simulink library "gasLibrary"  (R2019a)
settings: Solver=VariableStepAuto  StartTime=0.0  StopTime=10.0  RelTol=1e-3
values from neighbouring files (symbols this model uses):
  loadControlFlag = "on"    [gas_v1.m]
  loadState = "on"    [ColoradoGasModel.m]    (also in compressorTest.m = 'on'; experiment1.m = 'on'; experiment2.m = 'on'; experiment3.m = 'on')
  shutOffDuration = 3600    [ColoradoGasModel.m]
  shutOffPoint = 600    [ColoradoGasModel.m]
undefined symbols (not defined in the file or in its folder): f, powerSetPort, pressureSendPort, tempSendPort
libraries: fl_lib x48, nesl_utility x18, $bdroot x13, instrumentlib x5
settings Model: Creator=dzimm  LastModifiedBy=brandt

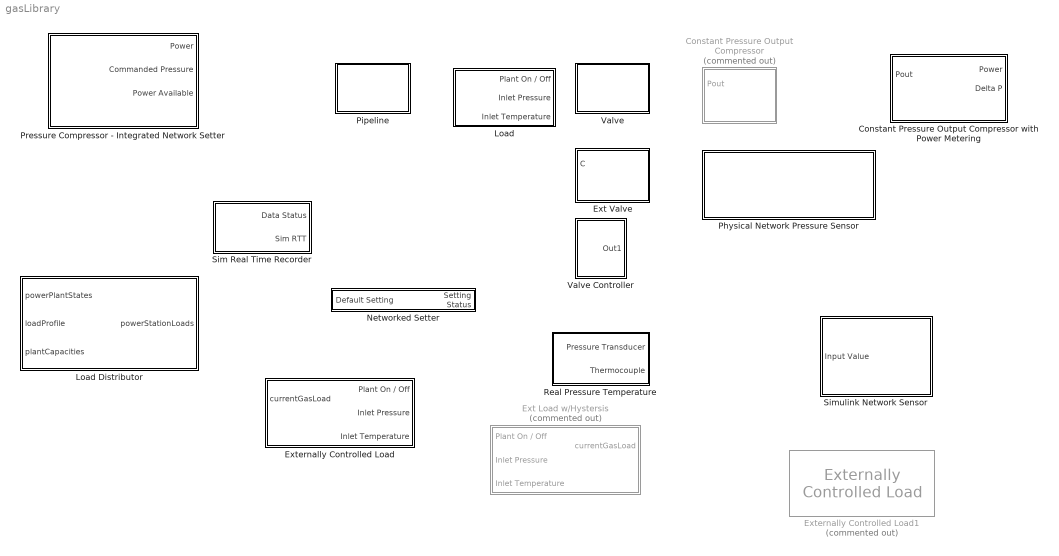
== system gasLibrary ==
  Constant Pressure Output Compressor : Subsystem  Commented=on  mask{xferNum=1, xferDen=[1800 1], delaySeconds=1, efficiency=0.3}
      mask prompts: xferNum "Plant Transfer Function Numerator (vector)"; xferDen "Plant Transfer Function Denominator (vector)"; delaySeconds "Response Delay (s)"; efficiency "Full Efficiency (-)"
  Constant Pressure Output Compressor with Power Metering : Subsystem  AncestorBlock=gasLibrary/Constant Pressure Output Compressor  mask{xferNum=1, xferDen=[1800 1], delaySeconds=1, efficiency=0.3, Numerator=[25]}
      mask prompts: xferNum "Plant Transfer Function Numerator (vector)"; xferDen "Plant Transfer Function Denominator (vector)"; delaySeconds "Response Delay (s)"; efficiency "Full Efficiency (-)"; Numerator "PSI Compression Ratio"
      mask TypeOptions Numerator: Power Transfer Function/Numerator
  Ext Load w/Hystersis : Subsystem  Commented=on  AncestorBlock=gasLibrary/Externally Controlled Load  mask{loadRow=0, loadState=loadState, pressureSendPort=8000, tempSendPort=9000, shutoff_duration=3600, shutoff_point=600}
      mask prompts: loadRow "Load Parameters (table row)"; loadState "Load Simulation Control ('on','off','initial')"; pressureSendPort "Pressure send port:"; tempSendPort "Temperature send port:"; shutoff_duration "Shut Off Duration (Seconds)"; shutoff_point "Shut Off Point (PSI)"
      mask init:
      | if(isempty(loadRow)||isnumeric(loadRow))
      |     loadName="Load";
      |     gasTime=[0 1e6]';
      |     gasLoad=[0 0]';
      |     textColor='red';
      |     pNominal=300;
      |     pCutoff=150;
      | else
      |     loadName=loadRow.Name;
      |     t=loadRow.Time{1};
      |     g=loadRow.Load{1};
      |     pNominal=loadRow.NominalPressure;
      |     pCutoff=loadRow.PressureCutoff;
      |     stopTime=loadRow.Time{1}(length(loadRow.Time{1}));
      |     switch(lower(loadState))
      |         case "on"
      | %             gasTime=t(:);
      | %             gasLoad=g(:);
      |             gasTime=[0 1e6]';
      |             gasLoad=[0 0]';
      |             textColor='green';
      |             loadFlag=[stopTime 1];
      |         case "off"
      |             textColor='red';
      |             gasTime=[0 1e6]';
      |             gasLoad=[0 0]';
      |             loadFlag=[stopTime 2];
      |         case "initial"
      |             textColor='blue';
      |             gasTime=[0 24*3600 1e6 ]';     % ramp gas on over one day
      |             gasLoad=[0 0       5   ]';     % gas ends at initial value
      |             loadFlag=[stopTime 3];
      |         otherwise
      |             fprintf("Cannot initialize\n");
      |             textColor='green';
      |     end
      | end
      mask TypeOptions pressureSendPort: Load Pressure UDP Send/Port
      mask TypeOptions tempSendPort: Load Temperature UDP Send/Port
      mask TypeOptions shutoff_duration: Pressure Shutoff/shutoff_duration
      mask TypeOptions shutoff_point: Pressure Shutoff/shutoff_point
      mask Display:
      | % tMax=max([gasTime(end)]);
      | set_param(gcb,'Name',loadName);
      | % color(textColor);
      | % text(0.1,0.8,sprintf("%s / %2.1f kg/s",loadState,max(gasLoad)))
      | % plot([0.2 0.8],[0.1 0.1]);
      | % plot([0.2 0.2],[0.1 0.6]);
      | % plot(gasTime/tMax*0.6+0.2,gasLoad/max(gasLoad)*0.5+0.1);
  Ext Valve : Subsystem  AncestorBlock=gasLibrary/Valve  mask{valveRow=[], valveState="on"}
      mask prompts: valveRow "Valve Control (table row)"; valveState "Valve Simulation Control ('on' 'off' 'initial')"
      mask init:
      | if(isempty(valveRow)||isnumeric(valveRow))
      |     valveName="Valve";
      |     valveTime=[0 1e6]';
      |     valveSetting=[0 0]';
      |     D=20;           % size of the valve
      |     Dmax=D-1;       % maximum port opening
      |     textColor='red';
      | else
      |     valveName=valveRow.Name;
      |     t=valveRow.Time{1};
      |     g=valveRow.State{1};
      |     D=valveRow.PortDiameter;
      |     Dmax=valveRow.MaxValveDiameter;
      |     switch(lower(valveState))
      |         case "on"
      |             valveTime=t(:);
      |             valveSetting=g(:);
      |             textColor='green';
      |         case "off"
      |             valveTime=[0 1e6]';
      |             valveSetting=[1 1]';
      |             textColor='red';
      |         case "initial"
      |             valveTime=[0 1e6 ]';   % ramp gas on over one day
      |             valveSetting=[g(1)    g(1)]';     % gas ends at initial value
      |             textColor='blue';
      |         otherwise
      |             fprintf("Cannot initialize\n");
      |             textColor='green';
      |     end
      | end
      mask Display:
      | set_param(gcb,'Name',valveName);
      | color(textColor);
      | if(valveState=="off")
      |     vLabel="bypass";
      | else
      |     vLabel="active";
      | end
      | text(0.1,0.8,sprintf("%s (%1d in)",vLabel,D))
      | plot([0.2 0.9],[0.3 0.3]);
      | plot([0.2 0.2],[0.1 0.6]);
      | plot(valveTime/max(valveTime)*0.65+0.2,double(valveSetting)*0.4+0.15);
  Externally Controlled Load : Subsystem  AncestorBlock=gasLibrary/Externally Controlled Load  mask{loadRow=0, loadState=loadState, pressureSendPort=8007, tempSendPort=8008, shutoff_duration=shutOffDuration, shutoff_point=shutOffPoint}
      mask prompts: loadRow "Load Parameters (table row)"; loadState "Load Simulation Control ('on','off','initial')"; pressureSendPort "Pressure send port:"; tempSendPort "Temperature send port:"; shutoff_duration "Shut Off Duration (Seconds)"; shutoff_point "Shut Off Point (PSI)"
      mask init: same as gasLibrary/Ext Load w/Hystersis
      mask TypeOptions pressureSendPort: Load Pressure UDP Send/Port
      mask TypeOptions tempSendPort: Load Temperature UDP Send/Port
      mask TypeOptions shutoff_duration: Pressure Shutoff/shutoff_duration
      mask TypeOptions shutoff_point: Pressure Shutoff/shutoff_point
      mask Display:
      | % tMax=max([gasTime(end)]);
      | set_param(gcb,'Name',loadName);
      | % color(textColor);
      | % text(0.1,0.8,sprintf("%s / %2.1f kg/s",loadState,max(gasLoad)))
      | % plot([0.2 0.8],[0.1 0.1]);
      | % plot([0.2 0.2],[0.1 0.6]);
      | % plot(gasTime/tMax*0.6+0.2,gasLoad/max(gasLoad)*0.5+0.1);
  Externally Controlled Load1 : $bdroot/Externally Controlled Load  Commented=on  loadRow=0  loadState=loadState  pressureSendPort=8007  tempSendPort=8008  shutoff_duration=shutoff_duration  shutoff_point=shutoff_point
  Load : Subsystem  mask{loadRow=0, loadState=loadControlFlag}
      mask prompts: loadRow "Load Parameters (table row)"; loadState "Load Simulation Control ('on','off','initial')"
      mask init:
      | if(isempty(loadRow)||isnumeric(loadRow))
      |     loadName="Load";
      |     gasTime=[0 1e6]';
      |     gasLoad=[0 0]';
      |     textColor='red';
      |     pNominal=300;
      |     pCutoff=150;
      | else
      |     loadName=loadRow.Name;
      |     t=loadRow.Time{1};
      |     g=loadRow.Load{1};
      |     pNominal=loadRow.NominalPressure;
      |     pCutoff=loadRow.PressureCutoff;
      |     switch(lower(loadState))
      |         case "on"
      |             gasTime=t(:);
      |             gasLoad=g(:);
      |             textColor='green';
      |         case "off"
      |             gasTime=[0 1e6]';
      |             gasLoad=[0 0]';
      |             textColor='red';
      |         case "initial"
      |             gasTime=[0 24*3600 1e6 ]';   % ramp gas on over one day
      |             gasLoad=[0 g(1)    g(1)]';     % gas ends at initial value
      |             textColor='blue';
      |         otherwise
      |             fprintf("Cannot initialize\n");
      |             textColor='green';
      |     end
      | end
      mask Display:
      | tMax=max([gasTime(end)]);
      | set_param(gcb,'Name',loadName);
      | color(textColor);
      | text(0.1,0.8,sprintf("%s / %2.1f kg/s",loadState,max(gasLoad)))
      | plot([0.2 0.8],[0.1 0.1]);
      | plot([0.2 0.2],[0.1 0.6]);
      | plot(gasTime/tMax*0.6+0.2,gasLoad/max(gasLoad)*0.5+0.1);
  Load Distributor : MATLAB Function  TreatAsAtomicUnit=on
  Networked Setter : Subsystem  mask{LocalPort=9090}
      mask prompts: LocalPort "Local port:"
      mask TypeOptions LocalPort: UDP Receive/LocalPort
  "Physical Network Pressure Sensor " : Subsystem
  Pipeline : Subsystem  mask{pipeRow=[]}
      mask prompts: pipeRow "Pipeilne Configuration (table row)"
      mask init:
      | if(isempty(pipeRow))
      |     pipeName="Pipeline";
      |     D=24;
      |     L=50;
      |     Pstart=300;
      | else
      |     pipeName=pipeRow.Name;
      |     D=pipeRow.DiameterInch;
      |     L=pipeRow.LengthMiles;
      |     Pstart=pipeRow.StartPressurePSI;
      | end
      mask Display:
      | fprintf('%1d"\n%1d miles\n%1d psi',D,L,Pstart)
      | set_param(gcb,'Name',pipeName)
  Pressure Compressor - Integrated Network Setter : Subsystem  AncestorBlock=gasLibrary/Constant Pressure Output Compressor  mask{xferNum=1, xferDen=[1800 1], delaySeconds=1, efficiency=0.3, pOutDefault=800, setterPort=9090, powerSetPort=powerSetPort, pressurePort=pressureSendPort, tempPort=tempSendPort}
      mask prompts: xferNum "Plant Transfer Function Numerator (vector)"; xferDen "Plant Transfer Function Denominator (vector)"; delaySeconds "Response Delay (s)"; efficiency "Full Efficiency (-)"; pOutDefault "Nominal Pressure:"; setterPort "Pressure setter port:"; powerSetPort "Power setter port:"; pressurePort "Pressure Port:"; tempPort "Temperature Port:"
      mask TypeOptions pOutDefault: Default POut/Value
      mask TypeOptions setterPort: Networked Setter/LocalPort
      mask TypeOptions powerSetPort: Max Power Setter/LocalPort
      mask TypeOptions pressurePort: Compressor Pressure UDP Send/Port
      mask TypeOptions tempPort: Compressor Temp UDP Send/Port
  Real Pressure Temperature : Subsystem  AncestorBlock=gasLibrary/Physical to Real Pressure Temperature
  Sim Real Time Recorder : Subsystem  mask{sendPort=6068, recPort=6065}
      mask prompts: sendPort "Send Port:"; recPort "Receive port:"
      mask TypeOptions sendPort: UDP Send/Port
      mask TypeOptions recPort: UDP Receive/LocalPort
  Simulink Network Sensor : Subsystem  mask{Port=7070}
      mask prompts: Port "Remote Port:"
      mask TypeOptions Port: UDP Send/Port
  Valve : Subsystem  mask{valveRow=[], valveState="on"}
      mask prompts: valveRow "Valve Control (table row)"; valveState "Valve Simulation Control ('on' 'off' 'initial')"
      mask init: same as gasLibrary/Ext Valve
      mask Display:
      | set_param(gcb,'Name',valveName);
      | color(textColor);
      | if(valveState=="off")
      |     vLabel="bypass";
      | else
      |     vLabel="active";
      | end
      | text(0.1,0.8,sprintf("%s (%1d in)",vLabel,D))
      | plot([0.2 0.9],[0.3 0.3]);
      | plot([0.2 0.2],[0.1 0.6]);
      | plot(valveTime/max(valveTime)*0.65+0.2,double(valveSetting)*0.4+0.15);
  Valve Controller : Subsystem

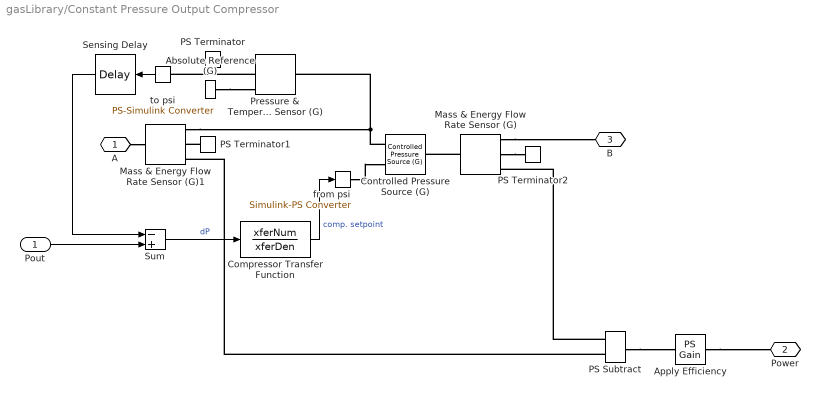
== system gasLibrary/Constant Pressure Output Compressor ==
  Pout : Inport
  Absolute Reference (G) : fl_lib/Gas/Elements/Absolute Reference (G)
      settings: SourceProductName=Simscape  SourceProductBaseCode=SS
  Apply Efficiency : fl_lib/Physical Signals/Functions/PS Gain  gain=1/efficiency
  Compressor Transfer Function : TransferFcn  Numerator=xferNum  Denominator=xferDen
  Controlled Pressure Source (G) : fl_lib/Gas/Sources/Controlled Pressure Source (G)  power_spec=1  area_A=24^2*pi/4 in^2  area_B=24^2*pi/4 in^2  mdot_A_specify=off  mdot_A_priority=None  mdot_A=1e-6 kg/s  mdot_A_nominal_specify=off  mdot_A_nominal_unit=kg/s  mdot_A_nominal_value=1
      settings: SourceProductName=Simscape  SourceProductBaseCode=SS
  Mass & Energy Flow Rate Sensor (G) : fl_lib/Gas/Sensors/Mass & Energy Flow Rate Sensor (G)
      settings: SourceProductName=Simscape  SourceProductBaseCode=SS
  Mass & Energy Flow Rate Sensor (G)1 : fl_lib/Gas/Sensors/Mass & Energy Flow Rate Sensor (G)
      settings: SourceProductName=Simscape  SourceProductBaseCode=SS
  PS Subtract : fl_lib/Physical Signals/Functions/PS Subtract
      settings: SourceProductName=Simscape
  PS Terminator : fl_lib/Physical Signals/Sinks/PS Terminator
      settings: SourceProductName=Simscape
  PS Terminator1 : fl_lib/Physical Signals/Sinks/PS Terminator
      settings: SourceProductName=Simscape
  PS Terminator2 : fl_lib/Physical Signals/Sinks/PS Terminator
      settings: SourceProductName=Simscape
  Pressure & Temperature Sensor (G) : fl_lib/Gas/Sensors/Pressure & Temperature Sensor (G)
      settings: SourceProductName=Simscape  SourceProductBaseCode=SS
  Sensing Delay : TransportDelay  DelayTime=delaySeconds  TransDelayFeedthrough=on
  Sum : Sum  Inputs=-+
  from psi : nesl_utility/Simulink-PS Converter  PhysicalDomain=network_engine_domain  SubClassName=ps_input  LeftPortType=input  RightPortType=output  PseudoPeriodic=off  Frequencies=[]  NoiseDistribution=none  NoiseParameters=[]  Unit=psi  AffineConversion=off  FilteringAndDerivatives=provide  SimscapeFilterOrder=1  InputFilterTimeConstant=0.001  UdotUserProvided=0
  to psi : nesl_utility/PS-Simulink Converter  PhysicalDomain=network_engine_domain  SubClassName=ps_output  LeftPortType=input  RightPortType=output  PseudoPeriodic=off  Frequencies=[]  Unit=psi  AffineConversion=off
  A : PMIOPort  Side=Left
  Power : PMIOPort  Port=2  Side=Right
  B : PMIOPort  Port=3  Side=Right
  wires:
  Pout/1 -> Sum/2
  Sum/1 -> Compressor Transfer Function/1  "dP"
  Compressor Transfer Function/1 -> from psi/1  "comp. setpoint"
  Sensing Delay/1 -> Sum/1
  to psi/1 -> Sensing Delay/1
  connections:
  Absolute Reference (G)/LConn1 -- Pressure & Temperature Sensor (G)/RConn1
  Pressure & Temperature Sensor (G)/RConn2 -- to psi/LConn1
  from psi/RConn1 -- Controlled Pressure Source (G)/LConn2
  PS Terminator/LConn1 -- Pressure & Temperature Sensor (G)/RConn3
  Controlled Pressure Source (G)/LConn1 -- Mass & Energy Flow Rate Sensor (G)1/RConn1 -- Pressure & Temperature Sensor (G)/LConn1
  Mass & Energy Flow Rate Sensor (G)/LConn1 -- Controlled Pressure Source (G)/RConn1
  Mass & Energy Flow Rate Sensor (G)/RConn1 -- B/RConn1
  A/RConn1 -- Mass & Energy Flow Rate Sensor (G)1/LConn1
  PS Terminator1/LConn1 -- Mass & Energy Flow Rate Sensor (G)1/RConn2
  Mass & Energy Flow Rate Sensor (G)/RConn2 -- PS Terminator2/LConn1
  PS Subtract/LConn1 -- Mass & Energy Flow Rate Sensor (G)/RConn3
  PS Subtract/LConn2 -- Mass & Energy Flow Rate Sensor (G)1/RConn3
  PS Subtract/RConn1 -- Apply Efficiency/LConn1
  Apply Efficiency/RConn1 -- Power/RConn1

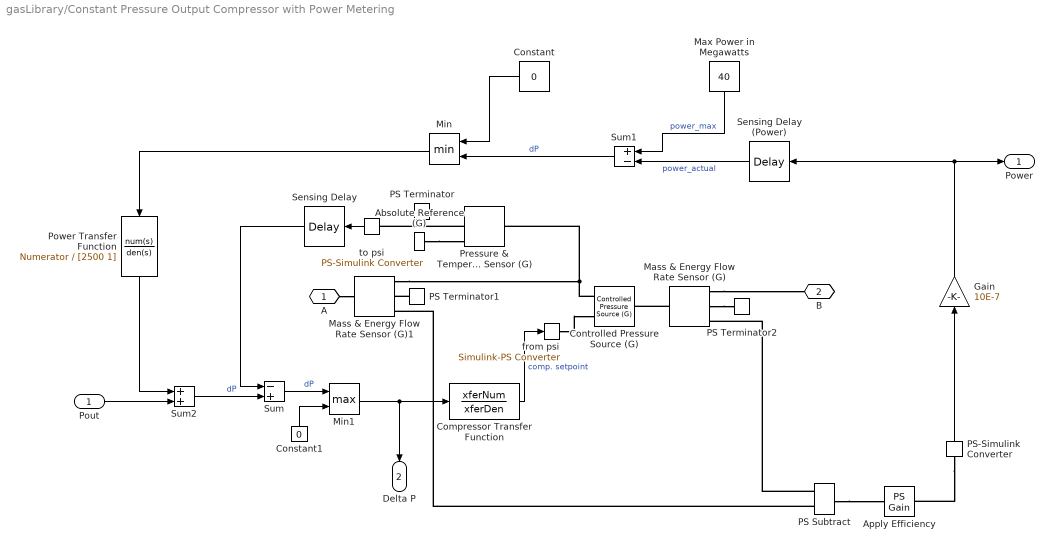
== system gasLibrary/Constant Pressure Output Compressor with Power Metering ==
  Pout : Inport
  Absolute Reference (G) : fl_lib/Gas/Elements/Absolute Reference (G)
      settings: SourceProductName=Simscape  SourceProductBaseCode=SS
  Apply Efficiency : fl_lib/Physical Signals/Functions/PS Gain  gain=1/efficiency
  Compressor Transfer Function : TransferFcn  Numerator=xferNum  Denominator=xferDen
  Constant : Constant  Value=0
  Constant1 : Constant  Value=0
  Controlled Pressure Source (G) : fl_lib/Gas/Sources/Controlled Pressure Source (G)  power_spec=1  area_A=24^2*pi/4 in^2  area_B=24^2*pi/4 in^2  mdot_A_specify=off  mdot_A_priority=None  mdot_A=1e-6 kg/s  mdot_A_nominal_specify=off  mdot_A_nominal_unit=kg/s  mdot_A_nominal_value=1
      settings: SourceProductName=Simscape  SourceProductBaseCode=SS
  Gain : Gain  Gain=10E-7
  Mass & Energy Flow Rate Sensor (G) : fl_lib/Gas/Sensors/Mass & Energy Flow Rate Sensor (G)
      settings: SourceProductName=Simscape  SourceProductBaseCode=SS
  Mass & Energy Flow Rate Sensor (G)1 : fl_lib/Gas/Sensors/Mass & Energy Flow Rate Sensor (G)
      settings: SourceProductName=Simscape  SourceProductBaseCode=SS
  Max Power in Megawatts : Constant  Value=40
  Min : MinMax  Inputs=2
  Min1 : MinMax  Function=max  Inputs=2
  PS Subtract : fl_lib/Physical Signals/Functions/PS Subtract
      settings: SourceProductName=Simscape
  PS Terminator : fl_lib/Physical Signals/Sinks/PS Terminator
      settings: SourceProductName=Simscape
  PS Terminator1 : fl_lib/Physical Signals/Sinks/PS Terminator
      settings: SourceProductName=Simscape
  PS Terminator2 : fl_lib/Physical Signals/Sinks/PS Terminator
      settings: SourceProductName=Simscape
  PS-Simulink Converter : nesl_utility/PS-Simulink Converter  PhysicalDomain=network_engine_domain  SubClassName=ps_output  LeftPortType=input  RightPortType=output  PseudoPeriodic=off  Frequencies=[]  Unit=W  AffineConversion=off
  Power Transfer Function : TransferFcn  Numerator=Numerator  Denominator=[2500 1]
  Pressure & Temperature Sensor (G) : fl_lib/Gas/Sensors/Pressure & Temperature Sensor (G)
      settings: SourceProductName=Simscape  SourceProductBaseCode=SS
  Sensing Delay : TransportDelay  DelayTime=delaySeconds  TransDelayFeedthrough=on
  Sensing Delay (Power) : TransportDelay  DelayTime=delaySeconds  TransDelayFeedthrough=on
  Sum : Sum  Inputs=-+
  Sum1 : Sum  Inputs=+-
  Sum2 : Sum
  from psi : nesl_utility/Simulink-PS Converter  PhysicalDomain=network_engine_domain  SubClassName=ps_input  LeftPortType=input  RightPortType=output  PseudoPeriodic=off  Frequencies=[]  NoiseDistribution=none  NoiseParameters=[]  Unit=psi  AffineConversion=off  FilteringAndDerivatives=provide  SimscapeFilterOrder=1  InputFilterTimeConstant=0.001  UdotUserProvided=0
  to psi : nesl_utility/PS-Simulink Converter  PhysicalDomain=network_engine_domain  SubClassName=ps_output  LeftPortType=input  RightPortType=output  PseudoPeriodic=off  Frequencies=[]  Unit=psi  AffineConversion=off
  A : PMIOPort  Side=Left
  B : PMIOPort  Port=2  Side=Right
  Power : Outport
  Delta P : Outport  Port=2
  wires:
  Compressor Transfer Function/1 -> from psi/1  "comp. setpoint"
  Sensing Delay/1 -> Sum/1
  to psi/1 -> Sensing Delay/1
  Sensing Delay (Power)/1 -> Sum1/2  "power_actual"
  Max Power in Megawatts/1 -> Sum1/1  "power_max"
  Sum1/1 -> Min/2  "dP"
  Constant/1 -> Min/1
  Min/1 -> Power Transfer Function/1
  Pout/1 -> Sum2/2
  PS-Simulink Converter/1 -> Gain/1
  Gain/1 -> Power/1, Sensing Delay (Power)/1
  Sum2/1 -> Sum/2  "dP"
  Sum/1 -> Min1/1  "dP"
  Min1/1 -> Delta P/1, Compressor Transfer Function/1
  Constant1/1 -> Min1/2
  Power Transfer Function/1 -> Sum2/1
  connections:
  Absolute Reference (G)/LConn1 -- Pressure & Temperature Sensor (G)/RConn1
  Pressure & Temperature Sensor (G)/RConn2 -- to psi/LConn1
  from psi/RConn1 -- Controlled Pressure Source (G)/LConn2
  PS Terminator/LConn1 -- Pressure & Temperature Sensor (G)/RConn3
  Controlled Pressure Source (G)/LConn1 -- Mass & Energy Flow Rate Sensor (G)1/RConn1 -- Pressure & Temperature Sensor (G)/LConn1
  Mass & Energy Flow Rate Sensor (G)/LConn1 -- Controlled Pressure Source (G)/RConn1
  Mass & Energy Flow Rate Sensor (G)/RConn1 -- B/RConn1
  A/RConn1 -- Mass & Energy Flow Rate Sensor (G)1/LConn1
  PS Terminator1/LConn1 -- Mass & Energy Flow Rate Sensor (G)1/RConn2
  Mass & Energy Flow Rate Sensor (G)/RConn2 -- PS Terminator2/LConn1
  PS Subtract/LConn1 -- Mass & Energy Flow Rate Sensor (G)/RConn3
  PS Subtract/LConn2 -- Mass & Energy Flow Rate Sensor (G)1/RConn3
  PS Subtract/RConn1 -- Apply Efficiency/LConn1
  PS-Simulink Converter/LConn1 -- Apply Efficiency/RConn1

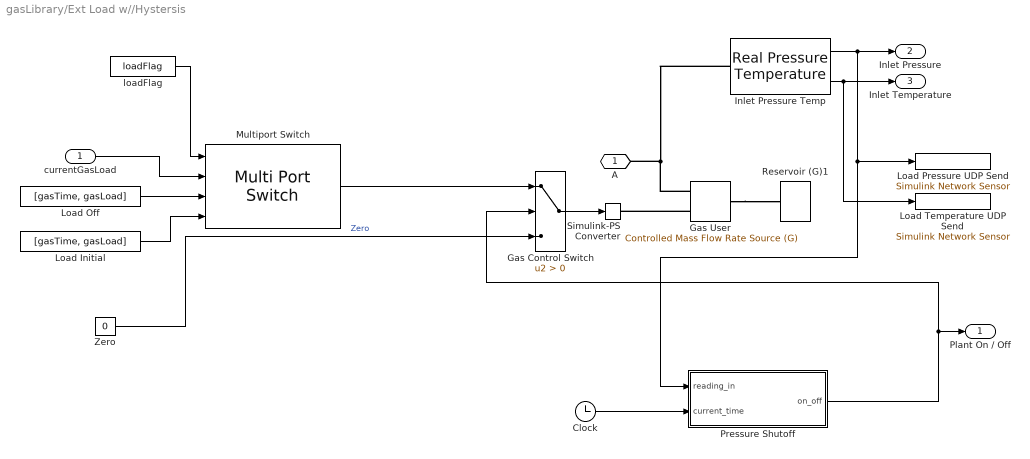
== system gasLibrary/Ext Load w//Hystersis ==
  currentGasLoad : Inport
  Clock : Clock
  Gas Control Switch : Switch  Criteria=u2 > Threshold
  Gas User : fl_lib/Gas/Sources/Controlled Mass Flow Rate Source (G)  power_spec=1  area_A=24^2*pi/4 in^2  area_B=20^2*pi/4 in^2  mdot_A_specify=on  mdot_A_priority=None  mdot_A=20 kg/s  mdot_A_nominal_specify=off  mdot_A_nominal_unit=kg/s  mdot_A_nominal_value=1
      settings: SourceProductName=Simscape  SourceProductBaseCode=SS
  Inlet Pressure Temp : $bdroot/Real Pressure Temperature  SystemSampleTime=-1
  Load Initial : FromWorkspace  VariableName=[gasTime, gasLoad]  SampleTime=0
  Load Off : FromWorkspace  VariableName=[gasTime, gasLoad]  SampleTime=0
  Load Pressure UDP Send : $bdroot/Simulink Network Sensor  Port=pressureSendPort
  Load Temperature UDP Send : $bdroot/Simulink Network Sensor  Port=tempSendPort
  Multiport Switch : MultiPortSwitch
  Pressure Shutoff : MATLAB Function  TreatAsAtomicUnit=on  SystemSampleTime=30  mask{shutoff_duration=shutoff_duration, shutoff_point=shutoff_point}
      mask prompts: shutoff_duration "Shut Off Duration (Seconds)"; shutoff_point "Shut Off Point (PSI)"
  Reservoir (G)1 : fl_lib/Gas/Elements/Reservoir (G)  pressure_spec=2  reservoir_pressure=300 psi  reservoir_temperature=25 degC  area_A=pi*25^2/4 in^2
      settings: SourceProductName=Foundation Library
  Simulink-PS Converter : nesl_utility/Simulink-PS Converter  PhysicalDomain=network_engine_domain  SubClassName=ps_input  LeftPortType=input  RightPortType=output  PseudoPeriodic=off  Frequencies=[]  NoiseDistribution=none  NoiseParameters=[]  Unit=1  AffineConversion=off  FilteringAndDerivatives=provide  SimscapeFilterOrder=1  InputFilterTimeConstant=0.001  UdotUserProvided=0
  Zero : Constant  Value=0
  loadFlag : FromWorkspace  VariableName=loadFlag  SampleTime=0
  A : PMIOPort  Side=Left
  Plant On / Off : Outport
  Inlet Pressure : Outport  Port=2
  Inlet Temperature : Outport  Port=3
  wires:
  Zero/1 -> Gas Control Switch/3  "Zero"
  Gas Control Switch/1 -> Simulink-PS Converter/1
  Multiport Switch/1 -> Gas Control Switch/1
  loadFlag/1 -> Multiport Switch/1
  Load Off/1 -> Multiport Switch/3
  Load Initial/1 -> Multiport Switch/4
  currentGasLoad/1 -> Multiport Switch/2
  Inlet Pressure Temp/1 -> Load Pressure UDP Send/1, Pressure Shutoff/1(reading_in), Inlet Pressure/1
  Inlet Pressure Temp/2 -> Load Temperature UDP Send/1, Inlet Temperature/1
  Clock/1 -> Pressure Shutoff/2(current_time)
  Pressure Shutoff/1(on_off) -> Gas Control Switch/2, Plant On / Off/1
  connections:
  Gas User/LConn2 -- Simulink-PS Converter/RConn1
  Inlet Pressure Temp/LConn1 -- A/RConn1 -- Gas User/LConn1
  Gas User/RConn1 -- Reservoir (G)1/LConn1

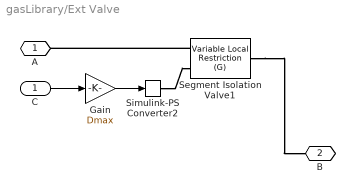
== system gasLibrary/Ext Valve ==
  C : Inport
  Gain : Gain  Gain=Dmax
  Segment Isolation Valve1 : fl_lib/Gas/Elements/Variable Local Restriction (G)  min_area=1e-4 in^2  max_area=pi*(Dmax-1)^2/4 in^2  area=pi*D^2/4 in^2  Cd=0.64  B_lam=0.999  mdot_A_specify=off  mdot_A_priority=None  mdot_A=1e-6 kg/s  mdot_A_nominal_specify=off  mdot_A_nominal_unit=kg/s  mdot_A_nominal_value=1
      settings: SourceProductName=Simscape  SourceProductBaseCode=SS
  Simulink-PS Converter2 : nesl_utility/Simulink-PS Converter  PhysicalDomain=network_engine_domain  SubClassName=ps_input  LeftPortType=input  RightPortType=output  PseudoPeriodic=off  Frequencies=[]  NoiseDistribution=none  NoiseParameters=[]  Unit=in^2  AffineConversion=off  FilteringAndDerivatives=provide  SimscapeFilterOrder=1  InputFilterTimeConstant=0.001  UdotUserProvided=0
  A : PMIOPort  Side=Left
  B : PMIOPort  Port=2  Side=Right
  wires:
  C/1 -> Gain/1
  Gain/1 -> Simulink-PS Converter2/1
  connections:
  Segment Isolation Valve1/RConn1 -- B/RConn1
  Segment Isolation Valve1/LConn1 -- A/RConn1
  Simulink-PS Converter2/RConn1 -- Segment Isolation Valve1/LConn2

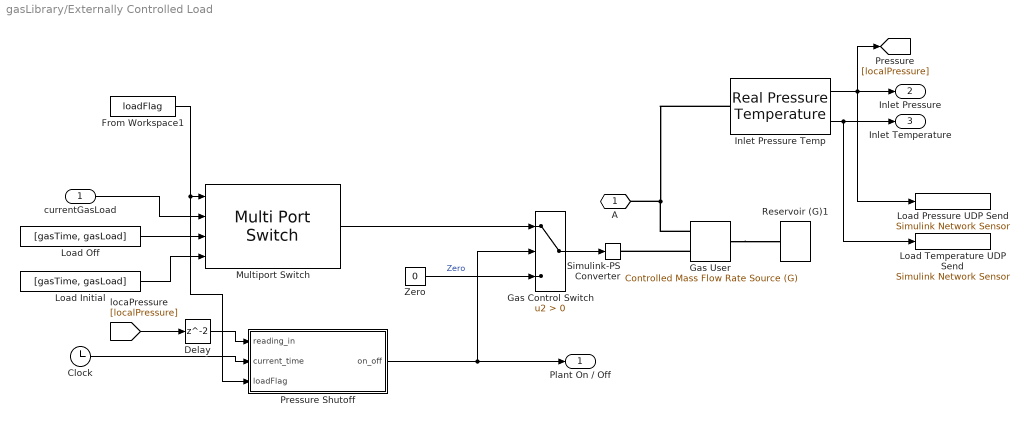
== system gasLibrary/Externally Controlled Load ==
  currentGasLoad : Inport
  Clock : Clock
  Delay : Delay
  From Workspace1 : FromWorkspace  VariableName=loadFlag  SampleTime=0
  Gas Control Switch : Switch  Criteria=u2 > Threshold
  Gas User : fl_lib/Gas/Sources/Controlled Mass Flow Rate Source (G)  power_spec=1  area_A=24^2*pi/4 in^2  area_B=20^2*pi/4 in^2  mdot_A_specify=on  mdot_A_priority=None  mdot_A=20 kg/s  mdot_A_nominal_specify=off  mdot_A_nominal_unit=kg/s  mdot_A_nominal_value=1
      settings: SourceProductName=Simscape  SourceProductBaseCode=SS
  Inlet Pressure Temp : $bdroot/Real Pressure Temperature  SystemSampleTime=-1
  Load Initial : FromWorkspace  VariableName=[gasTime, gasLoad]  SampleTime=0
  Load Off : FromWorkspace  VariableName=[gasTime, gasLoad]  SampleTime=0
  Load Pressure UDP Send : $bdroot/Simulink Network Sensor  Port=pressureSendPort
  Load Temperature UDP Send : $bdroot/Simulink Network Sensor  Port=tempSendPort
  Multiport Switch : MultiPortSwitch
  Pressure Shutoff : MATLAB Function  TreatAsAtomicUnit=on  SystemSampleTime=30  mask{shutoff_duration=shutoff_duration, shutoff_point=shutoff_point}
      mask prompts: shutoff_duration "Shut Off Duration (Seconds)"; shutoff_point "Shut Off Point (PSI)"
  Reservoir (G)1 : fl_lib/Gas/Elements/Reservoir (G)  pressure_spec=2  reservoir_pressure=300 psi  reservoir_temperature=25 degC  area_A=pi*25^2/4 in^2
      settings: SourceProductName=Foundation Library
  Simulink-PS Converter : nesl_utility/Simulink-PS Converter  PhysicalDomain=network_engine_domain  SubClassName=ps_input  LeftPortType=input  RightPortType=output  PseudoPeriodic=off  Frequencies=[]  NoiseDistribution=none  NoiseParameters=[]  Unit=1  AffineConversion=off  FilteringAndDerivatives=provide  SimscapeFilterOrder=1  InputFilterTimeConstant=0.001  UdotUserProvided=0
  Zero : Constant  Value=0
  A : PMIOPort  Side=Left
  Plant On / Off : Outport
  Inlet Pressure : Outport  Port=2
  Inlet Temperature : Outport  Port=3
  wires:
  Inlet Pressure Temp/2 -> Inlet Temperature/1, Load Temperature UDP Send/1
  Inlet Pressure Temp/1 -> [localPressure], Inlet Pressure/1, Load Pressure UDP Send/1
  currentGasLoad/1 -> Multiport Switch/2
  Load Initial/1 -> Multiport Switch/4
  Load Off/1 -> Multiport Switch/3
  From Workspace1/1 -> Pressure Shutoff/3(loadFlag), Multiport Switch/1
  Multiport Switch/1 -> Gas Control Switch/1
  Gas Control Switch/1 -> Simulink-PS Converter/1
  Clock/1 -> Pressure Shutoff/2(current_time)
  Pressure Shutoff/1(on_off) -> Gas Control Switch/2, Plant On / Off/1
  Zero/1 -> Gas Control Switch/3  "Zero"
  [localPressure] -> Delay/1
  Delay/1 -> Pressure Shutoff/1(reading_in)
  connections:
  Gas User/RConn1 -- Reservoir (G)1/LConn1
  Gas User/LConn1 -- A/RConn1 -- Inlet Pressure Temp/LConn1
  Gas User/LConn2 -- Simulink-PS Converter/RConn1

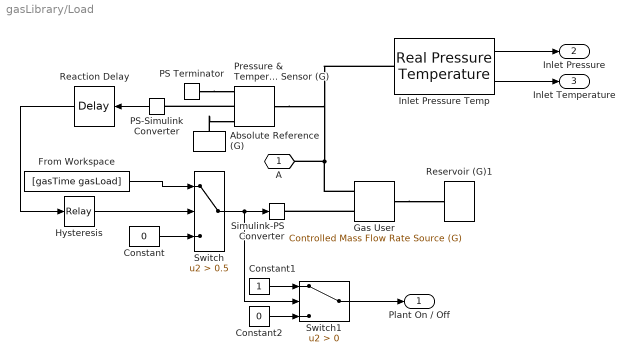
== system gasLibrary/Load ==
  Absolute Reference (G) : fl_lib/Gas/Elements/Absolute Reference (G)
      settings: SourceProductName=Simscape  SourceProductBaseCode=SS
  Constant : Constant  Value=0
  Constant1 : Constant
  Constant2 : Constant  Value=0
  From Workspace : FromWorkspace  VariableName=[gasTime gasLoad]  SampleTime=0  OutputAfterFinalValue=Holding final value
  Gas User : fl_lib/Gas/Sources/Controlled Mass Flow Rate Source (G)  power_spec=1  area_A=24^2*pi/4 in^2  area_B=20^2*pi/4 in^2  mdot_A_specify=on  mdot_A_priority=None  mdot_A=20 kg/s  mdot_A_nominal_specify=off  mdot_A_nominal_unit=kg/s  mdot_A_nominal_value=1
      settings: SourceProductName=Simscape  SourceProductBaseCode=SS
  Hysteresis : Relay  OnSwitchValue=pCutoff*1.05  OffSwitchValue=pCutoff
  Inlet Pressure Temp : $bdroot/Real Pressure Temperature  SystemSampleTime=-1
  PS Terminator : fl_lib/Physical Signals/Sinks/PS Terminator
      settings: SourceProductName=Simscape
  PS-Simulink Converter : nesl_utility/PS-Simulink Converter  PhysicalDomain=network_engine_domain  SubClassName=ps_output  LeftPortType=input  RightPortType=output  PseudoPeriodic=off  Frequencies=[]  Unit=psi  AffineConversion=off
  Pressure & Temperature Sensor (G) : fl_lib/Gas/Sensors/Pressure & Temperature Sensor (G)
      settings: SourceProductName=Simscape  SourceProductBaseCode=SS
  Reaction Delay : TransportDelay  DelayTime=60  InitialOutput=pNominal
  Reservoir (G)1 : fl_lib/Gas/Elements/Reservoir (G)  pressure_spec=2  reservoir_pressure=300 psi  reservoir_temperature=25 degC  area_A=pi*25^2/4 in^2
      settings: SourceProductName=Foundation Library
  Simulink-PS Converter : nesl_utility/Simulink-PS Converter  PhysicalDomain=network_engine_domain  SubClassName=ps_input  LeftPortType=input  RightPortType=output  PseudoPeriodic=off  Frequencies=[]  NoiseDistribution=none  NoiseParameters=[]  Unit=1  AffineConversion=off  FilteringAndDerivatives=provide  SimscapeFilterOrder=1  InputFilterTimeConstant=0.001  UdotUserProvided=0
  Switch : Switch  Criteria=u2 > Threshold  Threshold=0.5
  Switch1 : Switch  Criteria=u2 > Threshold
  A : PMIOPort  Side=Left
  Plant On / Off : Outport
  Inlet Pressure : Outport  Port=2
  Inlet Temperature : Outport  Port=3
  wires:
  Reaction Delay/1 -> Hysteresis/1
  PS-Simulink Converter/1 -> Reaction Delay/1
  Constant/1 -> Switch/3
  Hysteresis/1 -> Switch/2
  Switch/1 -> Switch1/2, Simulink-PS Converter/1
  Constant2/1 -> Switch1/3
  Switch1/1 -> Plant On / Off/1
  Constant1/1 -> Switch1/1
  Inlet Pressure Temp/1 -> Inlet Pressure/1
  Inlet Pressure Temp/2 -> Inlet Temperature/1
  From Workspace/1 -> Switch/1
  connections:
  Gas User/RConn1 -- Reservoir (G)1/LConn1
  Gas User/LConn1 -- Inlet Pressure Temp/LConn1 -- Pressure & Temperature Sensor (G)/LConn1 -- A/RConn1
  Gas User/LConn2 -- Simulink-PS Converter/RConn1
  PS Terminator/LConn1 -- Pressure & Temperature Sensor (G)/RConn3
  Absolute Reference (G)/LConn1 -- Pressure & Temperature Sensor (G)/RConn1
  Pressure & Temperature Sensor (G)/RConn2 -- PS-Simulink Converter/LConn1

== system gasLibrary/Networked Setter ==
  Default Setting : Inport
  Switch : Switch  Criteria=u2 > Threshold
  UDP Receive : instrumentlib/UDP Receive  Host=localhost  Port=4000  LocalPort=LocalPort  EnablePortSharing=off  GetLatestData=on  DataSize=[1 1]  DataType=double  ASCIIFormatting=%f,  Terminator=LF  ByteOrder=BigEndian  EnableBlockingMode=off  Timeout=10  SampleTime=300  LocalAddress=localhost
      settings: SourceProductName=Instrument Control Toolbox
  "Setting " : Outport
  Status : Outport  Port=2
  wires:
  Default Setting/1 -> Switch/3
  Switch/1 -> "Setting "/1
  UDP Receive/1 -> Switch/2, Switch/1
  UDP Receive/2 -> Status/1

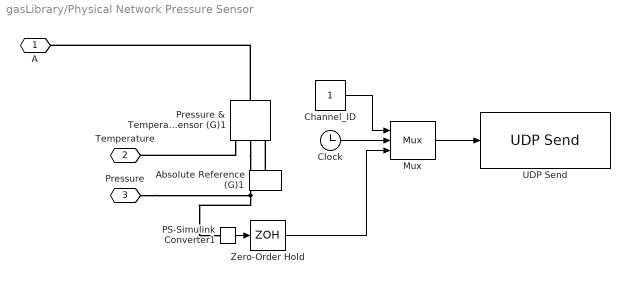
== system gasLibrary/Physical Network Pressure Sensor  ==
  Absolute Reference (G)1 : fl_lib/Gas/Elements/Absolute Reference (G)
      settings: SourceProductName=Simscape  SourceProductBaseCode=SS
  Channel_ID : Constant
  Clock : Clock
  Mux : Mux  Inputs=3
      settings: DisplayOption=signals
  PS-Simulink Converter1 : nesl_utility/PS-Simulink Converter  PhysicalDomain=network_engine_domain  SubClassName=ps_output  LeftPortType=input  RightPortType=output  PseudoPeriodic=off  Frequencies=[]  Unit=1  AffineConversion=off
  Pressure & Temperature Sensor (G)1 : fl_lib/Gas/Sensors/Pressure & Temperature Sensor (G)
      settings: SourceProductName=Simscape  SourceProductBaseCode=SS
  UDP Send : instrumentlib/UDP Send  Host=localhost  Port=7070  LocalPort=-1  EnablePortSharing=off  ByteOrder=BigEndian  OutputDatagramPacketSize=512  EnableBlockingMode=on  LocalAddress=0.0.0.0
      settings: SourceProductName=Instrument Control Toolbox
  Zero-Order Hold : ZeroOrderHold  SampleTime=300
  A : PMIOPort  Side=Left
  Temperature : PMIOPort  Port=2  Side=Right
  Pressure : PMIOPort  Port=3  Side=Right
  wires:
  PS-Simulink Converter1/1 -> Zero-Order Hold/1
  Zero-Order Hold/1 -> Mux/3
  Mux/1 -> UDP Send/1
  Clock/1 -> Mux/2
  Channel_ID/1 -> Mux/1
  connections:
  Absolute Reference (G)1/LConn1 -- Pressure & Temperature Sensor (G)1/RConn1
  Pressure & Temperature Sensor (G)1/RConn2 -- PS-Simulink Converter1/LConn1 -- Pressure/RConn1
  Pressure & Temperature Sensor (G)1/LConn1 -- A/RConn1
  Pressure & Temperature Sensor (G)1/RConn3 -- Temperature/RConn1

== system gasLibrary/Pipeline ==
  Line HT : fl_lib/Thermal/Thermal Elements/Conductive Heat Transfer  area=pi*(D/12)*(L*5280) ft^2  thickness=0.35 in  th_cond=54 W/(m*K)  T_specify=off  T_priority=None  T=0 K  T_nominal_specify=off  T_nominal_unit=K  T_nominal_value=1  Q_specify=off  Q_priority=None  Q=0 W  Q_nominal_specify=off  Q_nominal_unit=W  Q_nominal_value=1
      settings: SourceProductName=Simscape
  Pipe : fl_lib/Gas/Elements/Pipe (G)  length=L mi  area=D^2*pi/4 in^2  Dh=D in  length_add=100 ft  roughness=0.0018 in  Re_lam=2000  Re_tur=4000  shape_factor=64  Nu_lam=3.66  p_pipe_specify=on  p_pipe_priority=High  p_pipe=Pstart psi  p_pipe_nominal_specify=off  p_pipe_nominal_unit=MPa  p_pipe_nominal_value=1  T_pipe_specify=on  T_pipe_priority=High  T_pipe=25 degC  T_pipe_nominal_specify=off  T_pipe_nominal_unit=K  T_pipe_nominal_value=1  rho_pipe_specify=off  rho_pipe_priority=None  rho_pipe=14.4 kg/m^3  rho_pipe_nominal_specify=off  rho_pipe_nominal_unit=kg/m^3  rho_pipe_nominal_value=1
      settings: SourceProductName=Simscape  SourceProductBaseCode=SS
  Temperature Source : fl_lib/Thermal/Thermal Sources/Temperature Source  temperature=25 degC
      settings: SourceProductName=Simscape
  A : PMIOPort  Side=Left
  B : PMIOPort  Port=2  Side=Right
  connections:
  Pipe/RConn1 -- B/RConn1
  Pipe/LConn2 -- Line HT/RConn1
  Line HT/LConn1 -- Temperature Source/LConn1
  Pipe/LConn1 -- A/RConn1

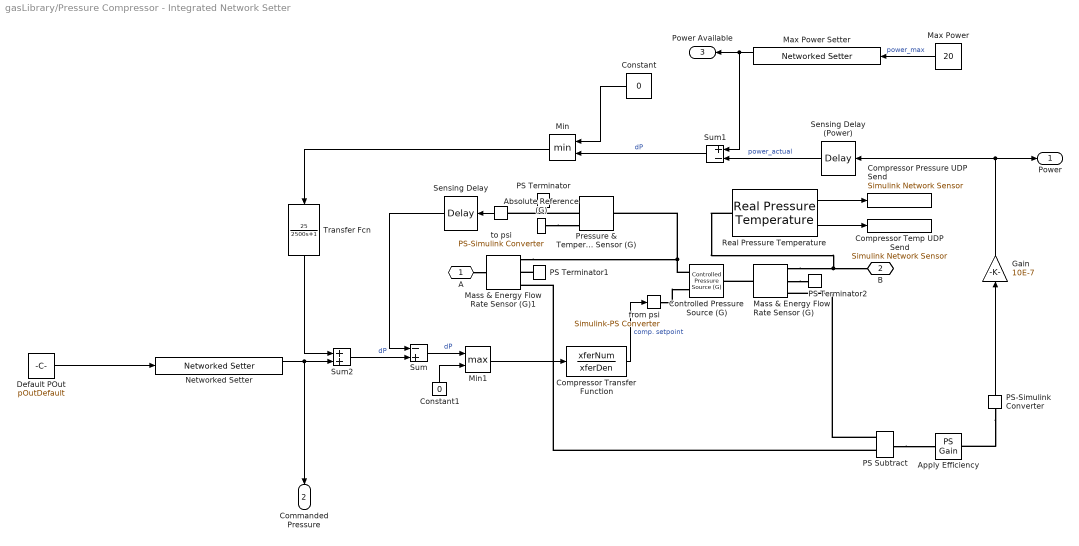
== system gasLibrary/Pressure Compressor - Integrated Network Setter ==
  Absolute Reference (G) : fl_lib/Gas/Elements/Absolute Reference (G)
      settings: SourceProductName=Simscape  SourceProductBaseCode=SS
  Apply Efficiency : fl_lib/Physical Signals/Functions/PS Gain  gain=1/efficiency
  Compressor Transfer Function : TransferFcn  Numerator=xferNum  Denominator=xferDen
  Compressor Pressure UDP Send : $bdroot/Simulink Network Sensor  Port=pressurePort
  Compressor Temp UDP Send : $bdroot/Simulink Network Sensor  Port=tempPort
  Constant : Constant  Value=0
  Constant1 : Constant  Value=0
  Controlled Pressure Source (G) : fl_lib/Gas/Sources/Controlled Pressure Source (G)  power_spec=1  area_A=24^2*pi/4 in^2  area_B=24^2*pi/4 in^2  mdot_A_specify=off  mdot_A_priority=None  mdot_A=1e-6 kg/s  mdot_A_nominal_specify=off  mdot_A_nominal_unit=kg/s  mdot_A_nominal_value=1
      settings: SourceProductName=Simscape  SourceProductBaseCode=SS
  Default POut : Constant  Value=pOutDefault
  Gain : Gain  Gain=10E-7
  Mass & Energy Flow Rate Sensor (G) : fl_lib/Gas/Sensors/Mass & Energy Flow Rate Sensor (G)
      settings: SourceProductName=Simscape  SourceProductBaseCode=SS
  Mass & Energy Flow Rate Sensor (G)1 : fl_lib/Gas/Sensors/Mass & Energy Flow Rate Sensor (G)
      settings: SourceProductName=Simscape  SourceProductBaseCode=SS
  Max Power : Constant  Value=20
  Max Power Setter : $bdroot/Networked Setter  LocalPort=powerSetPort
  Min : MinMax  Inputs=2
  Min1 : MinMax  Function=max  Inputs=2
  Networked Setter : $bdroot/Networked Setter  LocalPort=setterPort
  PS Subtract : fl_lib/Physical Signals/Functions/PS Subtract
      settings: SourceProductName=Simscape
  PS Terminator : fl_lib/Physical Signals/Sinks/PS Terminator
      settings: SourceProductName=Simscape
  PS Terminator1 : fl_lib/Physical Signals/Sinks/PS Terminator
      settings: SourceProductName=Simscape
  PS Terminator2 : fl_lib/Physical Signals/Sinks/PS Terminator
      settings: SourceProductName=Simscape
  PS-Simulink Converter : nesl_utility/PS-Simulink Converter  PhysicalDomain=network_engine_domain  SubClassName=ps_output  LeftPortType=input  RightPortType=output  PseudoPeriodic=off  Frequencies=[]  Unit=W  AffineConversion=off
  Pressure & Temperature Sensor (G) : fl_lib/Gas/Sensors/Pressure & Temperature Sensor (G)
      settings: SourceProductName=Simscape  SourceProductBaseCode=SS
  Real Pressure Temperature : $bdroot/Real Pressure Temperature  SystemSampleTime=-1
  Sensing Delay : TransportDelay  DelayTime=delaySeconds  TransDelayFeedthrough=on
  Sensing Delay (Power) : TransportDelay  DelayTime=delaySeconds  TransDelayFeedthrough=on
  Sum : Sum  Inputs=-+
  Sum1 : Sum  Inputs=+-
  Sum2 : Sum
  Transfer Fcn : TransferFcn  Numerator=[25]  Denominator=[2500 1]
  from psi : nesl_utility/Simulink-PS Converter  PhysicalDomain=network_engine_domain  SubClassName=ps_input  LeftPortType=input  RightPortType=output  PseudoPeriodic=off  Frequencies=[]  NoiseDistribution=none  NoiseParameters=[]  Unit=psi  AffineConversion=off  FilteringAndDerivatives=provide  SimscapeFilterOrder=1  InputFilterTimeConstant=0.001  UdotUserProvided=0
  to psi : nesl_utility/PS-Simulink Converter  PhysicalDomain=network_engine_domain  SubClassName=ps_output  LeftPortType=input  RightPortType=output  PseudoPeriodic=off  Frequencies=[]  Unit=psi  AffineConversion=off
  A : PMIOPort  Side=Left
  B : PMIOPort  Port=2  Side=Right
  Power : Outport
  Commanded Pressure : Outport  Port=2
  Power Available : Outport  Port=3
  wires:
  Compressor Transfer Function/1 -> from psi/1  "comp. setpoint"
  Sensing Delay/1 -> Sum/1
  to psi/1 -> Sensing Delay/1
  Sensing Delay (Power)/1 -> Sum1/2  "power_actual"
  Sum1/1 -> Min/2  "dP"
  Constant/1 -> Min/1
  Min/1 -> Transfer Fcn/1
  PS-Simulink Converter/1 -> Gain/1
  Gain/1 -> Power/1, Sensing Delay (Power)/1
  Sum2/1 -> Sum/2  "dP"
  Sum/1 -> Min1/1  "dP"
  Min1/1 -> Compressor Transfer Function/1
  Constant1/1 -> Min1/2
  Transfer Fcn/1 -> Sum2/1
  Default POut/1 -> Networked Setter/1
  Real Pressure Temperature/1 -> Compressor Pressure UDP Send/1
  Real Pressure Temperature/2 -> Compressor Temp UDP Send/1
  Networked Setter/1 -> Commanded Pressure/1, Sum2/2
  Max Power Setter/1 -> Power Available/1, Sum1/1
  Max Power/1 -> Max Power Setter/1  "power_max"
  connections:
  Absolute Reference (G)/LConn1 -- Pressure & Temperature Sensor (G)/RConn1
  Pressure & Temperature Sensor (G)/RConn2 -- to psi/LConn1
  from psi/RConn1 -- Controlled Pressure Source (G)/LConn2
  PS Terminator/LConn1 -- Pressure & Temperature Sensor (G)/RConn3
  Controlled Pressure Source (G)/LConn1 -- Pressure & Temperature Sensor (G)/LConn1 -- Mass & Energy Flow Rate Sensor (G)1/RConn1
  Mass & Energy Flow Rate Sensor (G)/LConn1 -- Controlled Pressure Source (G)/RConn1
  Mass & Energy Flow Rate Sensor (G)/RConn1 -- Real Pressure Temperature/LConn1 -- B/RConn1
  A/RConn1 -- Mass & Energy Flow Rate Sensor (G)1/LConn1
  PS Terminator1/LConn1 -- Mass & Energy Flow Rate Sensor (G)1/RConn2
  Mass & Energy Flow Rate Sensor (G)/RConn2 -- PS Terminator2/LConn1
  PS Subtract/LConn1 -- Mass & Energy Flow Rate Sensor (G)/RConn3
  PS Subtract/LConn2 -- Mass & Energy Flow Rate Sensor (G)1/RConn3
  PS Subtract/RConn1 -- Apply Efficiency/LConn1
  PS-Simulink Converter/LConn1 -- Apply Efficiency/RConn1

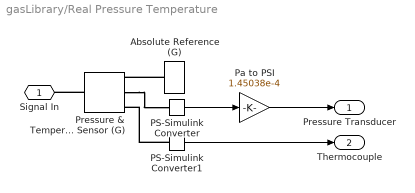
== system gasLibrary/Real Pressure Temperature ==
  Absolute Reference (G) : fl_lib/Gas/Elements/Absolute Reference (G)
      settings: SourceProductName=Simscape  SourceProductBaseCode=SS
  PS-Simulink Converter : nesl_utility/PS-Simulink Converter  PhysicalDomain=network_engine_domain  SubClassName=ps_output  LeftPortType=input  RightPortType=output  PseudoPeriodic=off  Frequencies=[]  Unit=1  AffineConversion=off
  PS-Simulink Converter1 : nesl_utility/PS-Simulink Converter  PhysicalDomain=network_engine_domain  SubClassName=ps_output  LeftPortType=input  RightPortType=output  PseudoPeriodic=off  Frequencies=[]  Unit=1  AffineConversion=off
  Pa to PSI : Gain  Gain=1.45038e-4
  Pressure & Temperature Sensor (G) : fl_lib/Gas/Sensors/Pressure & Temperature Sensor (G)
      settings: SourceProductName=Simscape  SourceProductBaseCode=SS
  Signal In : PMIOPort  Side=Left
  Pressure Transducer : Outport
  Thermocouple : Outport  Port=2
  wires:
  PS-Simulink Converter/1 -> Pa to PSI/1
  PS-Simulink Converter1/1 -> Thermocouple/1
  Pa to PSI/1 -> Pressure Transducer/1
  connections:
  Pressure & Temperature Sensor (G)/LConn1 -- Signal In/RConn1
  Absolute Reference (G)/LConn1 -- Pressure & Temperature Sensor (G)/RConn1
  PS-Simulink Converter1/LConn1 -- Pressure & Temperature Sensor (G)/RConn3
  Pressure & Temperature Sensor (G)/RConn2 -- PS-Simulink Converter/LConn1

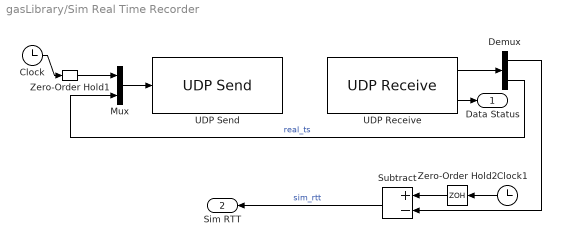
== system gasLibrary/Sim Real Time Recorder ==
  Clock : Clock
  Clock1 : Clock
  Demux : Demux  Outputs=2
  Mux : Mux  Inputs=2
  Subtract : Sum  Inputs=+-
  UDP Receive : instrumentlib/UDP Receive  Priority=2  Host=localhost  Port=6065  LocalPort=recPort  EnablePortSharing=off  GetLatestData=off  DataSize="[2  1]"  DataType=double  ASCIIFormatting=%f,  Terminator=LF  ByteOrder=BigEndian  EnableBlockingMode=off  Timeout=50  SampleTime=60  LocalAddress=localhost
      settings: SourceProductName=Instrument Control Toolbox
  UDP Send : instrumentlib/UDP Send  Priority=1  Host=localhost  Port=sendPort  LocalPort=-1  EnablePortSharing=off  ByteOrder=BigEndian  OutputDatagramPacketSize=24  EnableBlockingMode=on  LocalAddress=0.0.0.0
      settings: SourceProductName=Instrument Control Toolbox
  Zero-Order Hold1 : ZeroOrderHold  SampleTime=60
  Zero-Order Hold2 : ZeroOrderHold  SampleTime=-1
  Data Status : Outport
  Sim RTT : Outport  Port=2
  wires:
  Subtract/1 -> Sim RTT/1  "sim_rtt"
  Zero-Order Hold1/1 -> Mux/1
  Zero-Order Hold2/1 -> Subtract/1
  Mux/1 -> UDP Send/1
  UDP Receive/2 -> Data Status/1
  Demux/2 -> Mux/2  "real_ts"
  UDP Receive/1 -> Demux/1
  Demux/1 -> Subtract/2
  Clock/1 -> Zero-Order Hold1/1
  Clock1/1 -> Zero-Order Hold2/1

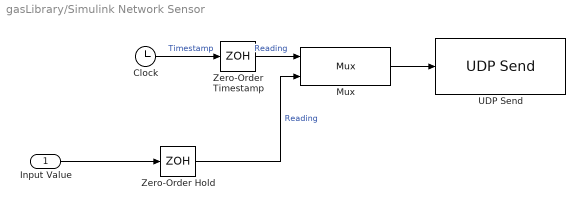
== system gasLibrary/Simulink Network Sensor ==
  Input Value : Inport
  Clock : Clock
  Mux : Mux  Inputs=2
      settings: DisplayOption=signals
  UDP Send : instrumentlib/UDP Send  Host=localhost  Port=Port  LocalPort=-1  EnablePortSharing=off  ByteOrder=BigEndian  OutputDatagramPacketSize=512  EnableBlockingMode=on  LocalAddress=0.0.0.0
      settings: SourceProductName=Instrument Control Toolbox
  Zero-Order Hold : ZeroOrderHold  SampleTime=300
  "Zero-Order Timestamp " : ZeroOrderHold  SampleTime=300
  wires:
  Input Value/1 -> Zero-Order Hold/1
  Zero-Order Hold/1 -> Mux/2  "Reading"
  Mux/1 -> UDP Send/1
  "Zero-Order Timestamp "/1 -> Mux/1  "Reading"
  Clock/1 -> "Zero-Order Timestamp "/1  "Timestamp"

== system gasLibrary/Valve ==
  From Workspace : FromWorkspace  VariableName=[valveTime valveSetting*Dmax]  SampleTime=0  OutputAfterFinalValue=Holding final value
  Segment Isolation Valve1 : fl_lib/Gas/Elements/Variable Local Restriction (G)  min_area=1e-4 in^2  max_area=pi*(Dmax-1)^2/4 in^2  area=pi*D^2/4 in^2  Cd=0.64  B_lam=0.999  mdot_A_specify=off  mdot_A_priority=None  mdot_A=1e-6 kg/s  mdot_A_nominal_specify=off  mdot_A_nominal_unit=kg/s  mdot_A_nominal_value=1
      settings: SourceProductName=Simscape  SourceProductBaseCode=SS
  Simulink-PS Converter2 : nesl_utility/Simulink-PS Converter  PhysicalDomain=network_engine_domain  SubClassName=ps_input  LeftPortType=input  RightPortType=output  PseudoPeriodic=off  Frequencies=[]  NoiseDistribution=none  NoiseParameters=[]  Unit=in^2  AffineConversion=off  FilteringAndDerivatives=provide  SimscapeFilterOrder=1  InputFilterTimeConstant=0.001  UdotUserProvided=0
  A : PMIOPort  Side=Left
  B : PMIOPort  Port=2  Side=Right
  wires:
  From Workspace/1 -> Simulink-PS Converter2/1
  connections:
  Segment Isolation Valve1/RConn1 -- B/RConn1
  Segment Isolation Valve1/LConn1 -- A/RConn1
  Simulink-PS Converter2/RConn1 -- Segment Isolation Valve1/LConn2

== system gasLibrary/Valve Controller ==
  Constant : Constant
  Constant1 : Constant  Value=0
  PS-Simulink Converter : nesl_utility/PS-Simulink Converter  PhysicalDomain=network_engine_domain  SubClassName=ps_output  LeftPortType=input  RightPortType=output  PseudoPeriodic=off  Frequencies=[]  Unit=1  AffineConversion=off
  Switch : Switch  Criteria=u2 > Threshold  Threshold=500
  A : PMIOPort  Side=Left
  Out1 : Outport
  wires:
  Constant1/1 -> Switch/3
  Switch/1 -> Out1/1
  Constant/1 -> Switch/1
  PS-Simulink Converter/1 -> Switch/2
  connections:
  A/RConn1 -- PS-Simulink Converter/LConn1

== matlab function gasLibrary/Ext Load w//Hystersis/Pressure Shutoff ==
  data: reading_in input; on_off output; current_time input; shutoff_duration parameter; shutoff_point parameter
function on_off = fcn(reading_in, current_time, shutoff_duration, shutoff_point)

persistent shut_off_time;
persistent state;
if (isempty(shut_off_time))
    shut_off_time=0;
    state=1;
end

% currently running
if state == 1 
    if reading_in < shutoff_point
         on_off = 0;
         shut_off_time = current_time;
         state = 0;
    end
% currently off
else
    if current_time > shut_off_time + shutoff_duration
        on_off = 1;
        state = 1;
    end
end

== matlab function gasLibrary/Load Distributor ==
  data: powerPlantStates input; powerStationLoads output; loadProfile input; plantCapacities input
function powerStationLoads = fcn(powerPlantStates, loadProfile, plantCapacities)
powerPlantStates=powerPlantStates==1;
totalCapacity=sum(powerPlantStates .* plantCapacities);
loadProfile=min(loadProfile, totalCapacity);
loadFractions=(powerPlantStates .* plantCapacities) / totalCapacity;
powerStationLoads=loadFractions*loadProfile;

== matlab function gasLibrary/Externally Controlled Load/Pressure Shutoff ==
  data: reading_in input; on_off output; current_time input; loadFlag input; shutoff_duration parameter; shutoff_point parameter
function on_off = fcn(reading_in, current_time, loadFlag, shutoff_duration, shutoff_point)

persistent shut_off_time;
persistent state;
persistent stochastic_shutoff;

if (isempty(shut_off_time))
    shut_off_time=0;
    state=1;
    stochastic_shutoff=shutoff_duration+(rand*shutoff_duration);
end

on_off=state;

% currently running
if state == 1
    if (reading_in < shutoff_point) && (loadFlag == 1) && (current_time > 3600)
         on_off = 0;
         shut_off_time = current_time;
         state = 0;
    end
% currently off
else
    if current_time > shut_off_time + stochastic_shutoff
        on_off = 1;
        state = 1;
    end
end
